simulink model "Prob_8_model"  (R2016a)
settings: Solver=VariableStepAuto  StartTime=0.0  StopTime=10.0  RelTol=1e-3
settings Model: Creator=Admin  LastModifiedBy=Admin

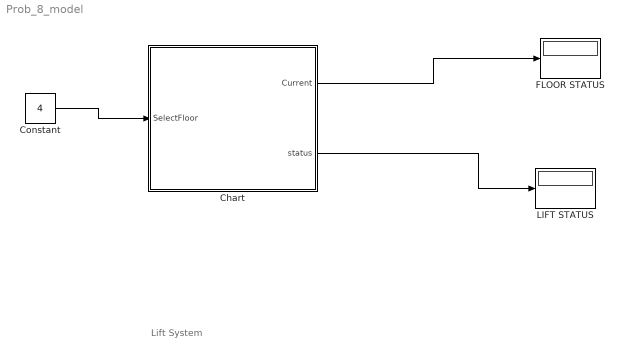
== system Prob_8_model ==
  note: Lift System
  Chart : Stateflow chart  TreatAsAtomicUnit=on
  Constant : Constant  Value=4
  "FLOOR STATUS " : Display
  "LIFT STATUS " : Display
  wires:
  Chart/2(status) -> "LIFT STATUS "/1
  Constant/1 -> Chart/1(SelectFloor)
  Chart/1(Current) -> "FLOOR STATUS "/1

== stateflow chart Prob_8_model/Chart ==
  state LiftOperation [parallel]
    entry:
    status=0;
    settings: executionOrder=1
    state LiftOn
      state GroundFloor
        entry:
        status=1;
        during:
        Current=0;
        CheckFloor(Current);
        exit:
        status=0;
      state FirstFloor
        entry:
        status=1;
        during:
        Current=1;
        CheckFloor(Current);
        exit:
        status=0;
      state SecondFloor
        entry:
        status=1;
        during:
        Current=2;
        CheckFloor(Current);
        exit:
        status=0;
      state ThirdFloor
        entry:
        status=1;
        during:
        Current=3;
        CheckFloor(Current);
        exit:
        status=0;
      state FourthFloor
        entry:
        status=1
        during:
        Current=4;
        CheckFloor(Current);
        exit:
        status=0;
      state FifthFloor
        entry:
        status=1;
        during:
        Current=5;
        CheckFloor(Current);
        exit:
        status=0;
      (default) -> GroundFloor
      GroundFloor -> FirstFloor : up
      FirstFloor -> GroundFloor [order 2] : down
      FirstFloor -> SecondFloor [order 1] : up
      SecondFloor -> FirstFloor [order 2] : down
      SecondFloor -> ThirdFloor [order 1] : up
      ThirdFloor -> SecondFloor [order 2] : down
      ThirdFloor -> FourthFloor [order 1] : up
      FourthFloor -> ThirdFloor [order 1] : down
      FourthFloor -> FifthFloor [order 2] : up
      FifthFloor -> FourthFloor : down
    (default) -> LiftOn
  state y = CheckFloor(Floor) [function]
    (default) -> (junction 91)
    (junction 91) -> (junction 88) [order 3] : [SelectFloor<Floor]{
        | send(down);
        | disp('LiftMovingDown');}
    (junction 91) -> (junction 96) [order 1] : [SelectFloor>Floor]{
        | send(up);
        | disp('LiftMovingUp');}
    (junction 88) -> (junction 97)
    (junction 91) -> (junction 85) [order 2] : [SelectFloor==Floor]{
        | disp('Current');}
    (junction 96) -> (junction 93)
    (junction 97) -> (junction 85)
    (junction 93) -> (junction 85)
    (junction 85) -> (junction 92)
  data: Floor function_input; y function_output; SelectFloor input; Current output; status output; alarmStatus local
  events: down local FUNCTION_CALL_EVENT; up local FUNCTION_CALL_EVENT; off local FUNCTION_CALL_EVENT; on local FUNCTION_CALL_EVENT
